simulink model "teste"  (R2017a)
settings: Solver=VariableStepAuto  StartTime=0.0  StopTime=10.0  RelTol=1e-3
settings Model: Creator=felip  LastModifiedBy=felip

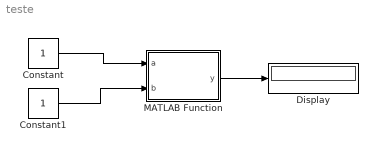
== system teste ==
  Constant : Constant
  Constant1 : Constant
  Display : Display
  MATLAB Function : MATLAB Function  TreatAsAtomicUnit=on
  wires:
  Constant/1 -> MATLAB Function/1(a)
  Constant1/1 -> MATLAB Function/2(b)
  MATLAB Function/1(y) -> Display/1

== matlab function teste/MATLAB Function ==
  data: a input; y output; b input
function y = fcn(a, b)
coder.extrinsic('solveSyms');
y=0;
y = solveSyms(a,b);
